simulink model "teleoperation_2017a"  (R2018a)
settings: Solver=ode45  StartTime=0.0  StopTime=1000  FixedStep=0.001  RelTol=1e-3
values from neighbouring files (symbols this model uses):
  B_e = 0.01    [Teleop.m]
  B_h = 4.0    (= 4)    [Teleop.m]
  B_v = 0.44    [Teleop.m]
  J_m = 0.0001    [Teleop.m]
  J_s = 0.0001    [Teleop.m]
  J_v = 0.0007    [Teleop.m]
  K_h = 200.0    (= 200)    [Teleop.m]
  K_v = 20.0    (= 20)    [Teleop.m]
settings Model: Creator=blue_orangotan  LastModifiedBy=blue_orangotan
settings CodeAppCC: StateflowObjectComments=on

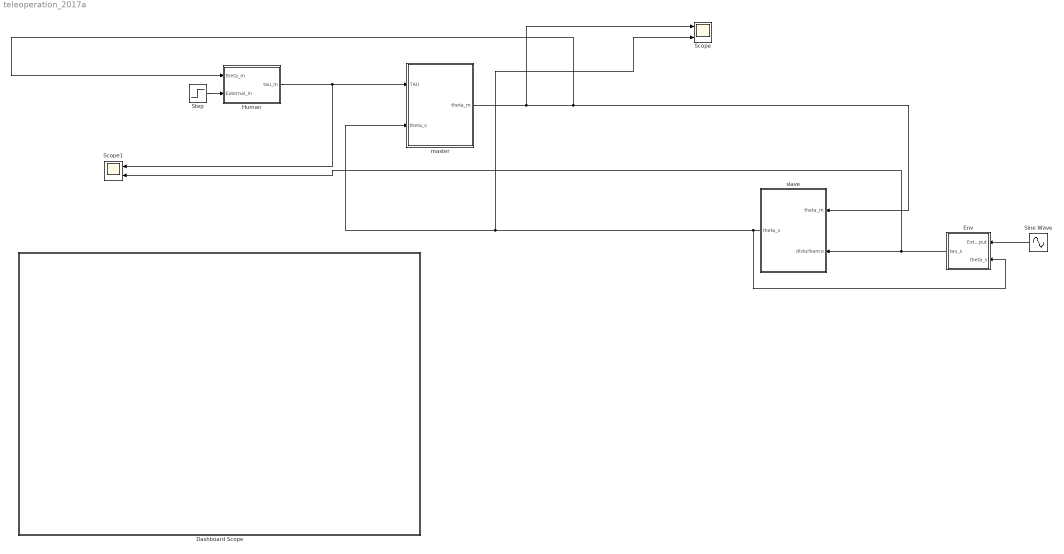
== system teleoperation_2017a ==
  Dashboard Scope : Subsystem  DialogController=hmiCreateDDGDialog  IsWebBlock=on  mask(MWDashboardBlock){webBlockId=d953983e-eab8-4310-ba24-9145e9f5b59c, webBlockType=sdiscope, ShowInitialText=on, HMISrcModelName=teleoperation_2017a}
      mask prompts: webBlockId "WebBlock Id"; webBlockType "WebBlock Type"; HMISrcModelName "Source Model"
      mask help: SimulinkHMI:dialogs:HMIScopeDialogDesc
      mask Help: helpview([docroot '/mapfiles/simulink.map'], 'hmi_scope')
      mask Display:
      | if strcmp(get_param(bdroot(gcb),'BlockDiagramType'), 'library')
      |     image([(matlabroot) '/toolbox/simulink/hmi/icons/DashboardScope.png']);
      | end
  Env : Subsystem
  Human : Subsystem
  Scope : Scope  NumInputPorts=3
  Scope1 : Scope  NumInputPorts=2
  Sine Wave : Sin  SampleTime=0
  Step : Step  SampleTime=0
  master : Subsystem
  "slave " : Subsystem
  wires:
  master/1(theta_m) -> Scope/1, Human/1(theta_m), "slave "/1("theta_m ")
  "slave "/1(theta_s) -> Scope/3, master/2(theta_s), Env/2(theta_s)
  Sine Wave/1 -> Env/1(External_input)
  Env/1("tau_s ") -> Scope1/2, "slave "/2(disturbance)
  Step/1 -> Human/2(External_in)
  Human/1(tau_m) -> Scope1/1, master/1(TAU)

== system teleoperation_2017a/Dashboard Scope ==

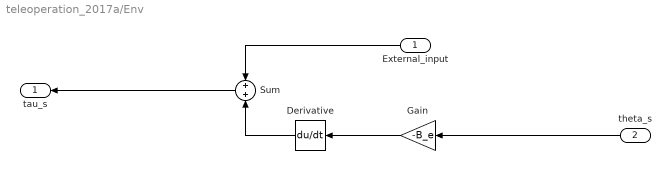
== system teleoperation_2017a/Env ==
  External_input : Inport
  theta_s : Inport  Port=2
  Derivative : Derivative  CoefficientInTFapproximation=0
  Gain : Gain  Gain=-B_e
  Sum : Sum
  "tau_s " : Outport
  wires:
  External_input/1 -> Sum/1
  theta_s/1 -> Gain/1
  Gain/1 -> Derivative/1
  Derivative/1 -> Sum/2
  Sum/1 -> "tau_s "/1

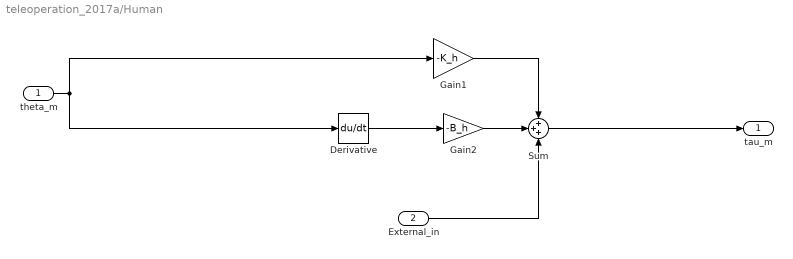
== system teleoperation_2017a/Human ==
  theta_m : Inport
  External_in : Inport  Port=2
  Derivative : Derivative  CoefficientInTFapproximation=0
  Gain1 : Gain  Gain=-K_h
  Gain2 : Gain  Gain=-B_h
  Sum : Sum  Inputs=+++
  tau_m : Outport
  wires:
  Derivative/1 -> Gain2/1
  theta_m/1 -> Gain1/1, Derivative/1
  Sum/1 -> tau_m/1
  Gain2/1 -> Sum/2
  Gain1/1 -> Sum/1
  External_in/1 -> Sum/3

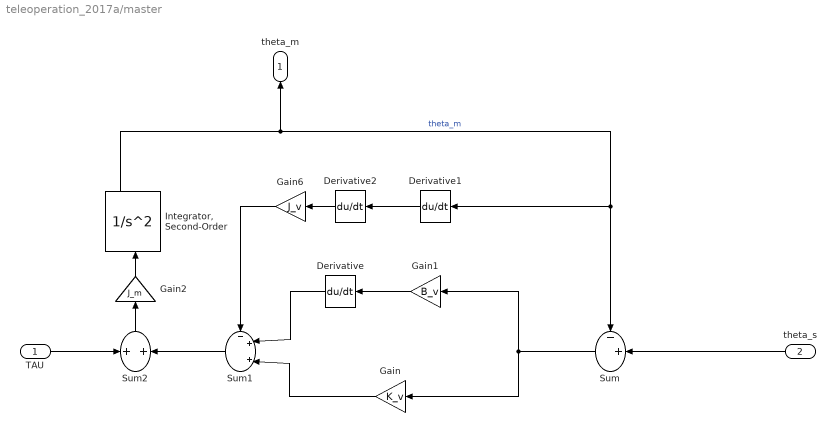
== system teleoperation_2017a/master ==
  TAU : Inport
  theta_s : Inport  Port=2
  Derivative : Derivative  CoefficientInTFapproximation=0
  Derivative1 : Derivative  CoefficientInTFapproximation=0
  Derivative2 : Derivative  CoefficientInTFapproximation=0
  Gain : Gain  Gain=K_v
  Gain1 : Gain  Gain=B_v
  Gain2 : Gain  Gain=J_m
  Gain6 : Gain  Gain=J_v
  "Integrator, Second-Order" : SecondOrderIntegrator  ICX=0
  Sum : Sum  Inputs=-+|
  Sum1 : Sum  Inputs=-++|
  Sum2 : Sum  Inputs=+|+
  theta_m : Outport
  wires:
  Derivative1/1 -> Derivative2/1
  "Integrator, Second-Order"/1 -> theta_m/1, Derivative1/1, Sum/1  "theta_m"
  theta_s/1 -> Sum/2
  Gain/1 -> Sum1/3
  Sum/1 -> Gain/1, Gain1/1
  Sum1/1 -> Sum2/2
  Derivative2/1 -> Gain6/1
  Derivative/1 -> Sum1/2
  Gain6/1 -> Sum1/1
  Gain1/1 -> Derivative/1
  Sum2/1 -> Gain2/1
  Gain2/1 -> "Integrator, Second-Order"/1
  TAU/1 -> Sum2/1

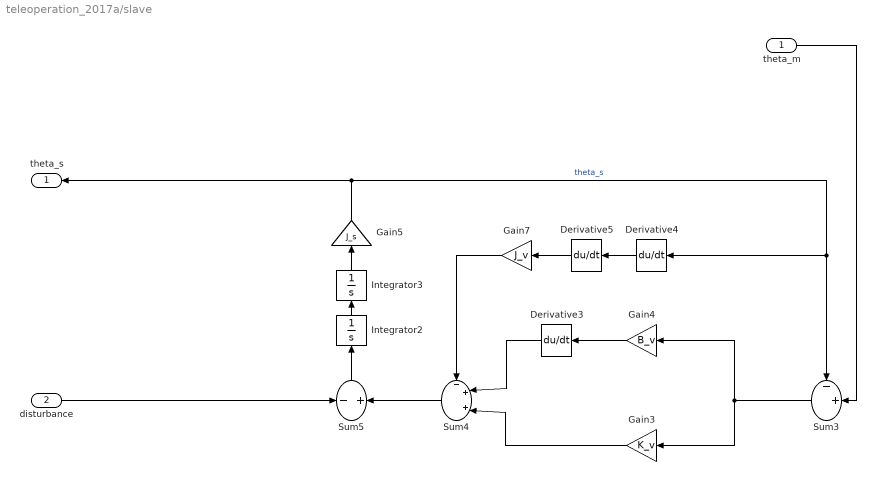
== system teleoperation_2017a/slave  ==
  "theta_m " : Inport
  disturbance : Inport  Port=2
  Derivative3 : Derivative  CoefficientInTFapproximation=0
  Derivative4 : Derivative  CoefficientInTFapproximation=0
  Derivative5 : Derivative  CoefficientInTFapproximation=0
  Gain3 : Gain  Gain=K_v
  Gain4 : Gain  Gain=B_v
  Gain5 : Gain  Gain=J_s
  Gain7 : Gain  Gain=J_v
  Integrator2 : Integrator
  Integrator3 : Integrator
  Sum3 : Sum  Inputs=-+|
  Sum4 : Sum  Inputs=-++|
  Sum5 : Sum  Inputs=-|+
  theta_s : Outport
  wires:
  Sum5/1 -> Integrator2/1
  Gain7/1 -> Sum4/1
  Integrator3/1 -> Gain5/1
  Integrator2/1 -> Integrator3/1
  Derivative5/1 -> Gain7/1
  Sum4/1 -> Sum5/2
  Derivative3/1 -> Sum4/2
  Gain4/1 -> Derivative3/1
  Gain5/1 -> theta_s/1, Derivative4/1, Sum3/1  "theta_s"
  Gain3/1 -> Sum4/3
  "theta_m "/1 -> Sum3/2
  Sum3/1 -> Gain3/1, Gain4/1
  Derivative4/1 -> Derivative5/1
  disturbance/1 -> Sum5/1
